simulink model "estimExp"  (R2017a)
settings: Solver=FixedStepDiscrete  StartTime=0.0  StopTime=20  FixedStep=prms.Ts  RelTol=1e-3
undefined symbols (not defined in the file or in its folder): prms
libraries: raspi_library x5, simulink x2
settings Model: SimulationMode=external  Creator=The MathWorks Inc.  LastModifiedBy=marti
settings SolverCC: PositivePriorityOrder=on
settings DataIOCC: LimitDataPoints=on  SaveFormat=Array
settings OptimizationCC: BlockReduction=off  BooleanDataType=off  DefaultUnderspecifiedDataType=single  LifeSpan=inf  MaxStackSize=64
settings DebuggingCC: SaveWithParameterizedLinksMsg=none  UnderspecifiedInitializationDetection=Classic  MergeDetectMultiDrivingBlocksExec=none  SignalResolutionControl=TryResolveAllWithWarning  InheritedTsInSrcMsg=error  ParameterTunabilityLossMsg=error  SFUnexpectedBacktrackingDiag=warning  SFNoUnconditionalDefaultTransitionDiag=warning  SFExecutionAtInitializationDiag=none
settings HardwareCC: ProdBitPerPointer=32  ProdBitPerSizeT=32  ProdBitPerPtrDiffT=32  ProdLargestAtomicInteger=Long  ProdLargestAtomicFloat=Double  ProdWordSize=32  ProdHWDeviceType=ARM Compatible->ARM Cortex
settings ModelReferenceCC: PropagateSignalLabelsOutOfModel=off
settings SFSimCC: MATLABDynamicMemAlloc=off
settings RTWCC: SystemTargetFile=ert.tlc  HardwareBoard=Raspberry Pi  TLCOptions=-aInlineSetEventsForThisBaseRateFcn=TLC_FALSE -aSuppressMultiTaskScheduler=TLC_FALSE -aRateBasedStepFcn=0  TemplateMakefile=ert_default_tmf  Description=Embedded Coder  GenerateReport=on  RTWVerbose=off  Toolchain=GNU GCC Raspberry Pi  BuildConfiguration=Specify  IncludeHyperlinkInReport=on  GenerateTraceInfo=on  GenerateTraceReport=on  GenerateTraceReportSl=on  GenerateTraceReportSf=on  GenerateTraceReportEml=on
settings CodeAppCC: ForceParamTrailComments=on  IgnoreCustomStorageClasses=off  OperatorAnnotations=on  SimulinkDataObjDesc=on  SFDataObjDesc=on  MATLABFcnDesc=on  MangleLength=10  InsertBlockDesc=on  MATLABSourceComments=on
settings ERTTargetCC: MultiwordLength=2048  SupportContinuousTime=on  SupportVariableSizeSignals=on
settings ConfigComp: CovMetricSettings=dw  CovHtmlReporting=on  CovSaveCumulativeToWorkspaceVar=on  CovSaveSingleToWorkspaceVar=on  CovExternalEMLEnable=off  CovSFcnEnable=off

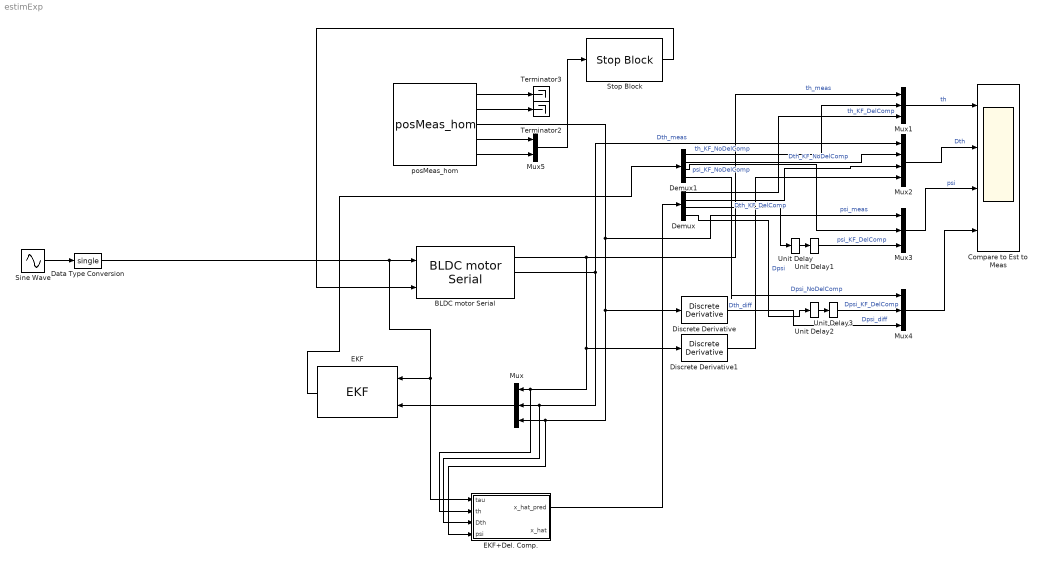
== system estimExp ==
  BLDC motor Serial : raspi_library/BLDC motor Serial  sampleTime=prms.Ts
  Compare to Est to Meas : Scope  NumInputPorts=4
  Data Type Conversion : DataTypeConversion  OutDataTypeStr=single
  Demux : Demux
  Demux1 : Demux
  Discrete Derivative : simulink/Discrete/Discrete Derivative  gainval=1.0  ICPrevScaledInput=0.0  OutMin=[]  OutMax=[]  OutDataType=fixdt(1, 16)  OutScaling=2^-10  DoSatur=off
  Discrete Derivative1 : simulink/Discrete/Discrete Derivative  gainval=1.0  ICPrevScaledInput=0.0  OutMin=[]  OutMax=[]  OutDataType=fixdt(1, 16)  OutScaling=2^-10  DoSatur=off
  EKF : raspi_library/EKF
  EKF+Del. Comp. : Subsystem
  Mux{,1,3..4} (4 alike) : Mux  Inputs=3
  Mux2 : Mux
  Mux5 : Mux  Inputs=2
  Sine Wave : Sin  Amplitude=0.05  Frequency=2*pi  SampleTime=prms.Ts
  Stop Block : raspi_library/Stop Block
  Terminator2 : Terminator
  Terminator3 : Terminator
  Unit Delay{,1..3} (4 alike) : UnitDelay  SampleTime=-1
  posMeas_hom : raspi_library/posMeas_hom  H=H  sampleTime=prms.Ts
  wires:
  posMeas_hom/5 -> Mux5/2
  posMeas_hom/4 -> Mux5/1
  posMeas_hom/2 -> Terminator2/1
  posMeas_hom/1 -> Terminator3/1
  posMeas_hom/3 -> Mux3/1, Discrete Derivative/1, EKF+Del. Comp./4(psi), Mux/3  "psi_meas"
  Mux/1 -> EKF/2
  BLDC motor Serial/1 -> Discrete Derivative1/1, EKF+Del. Comp./2(th), Mux/1, Mux1/1  "th_meas"
  BLDC motor Serial/2 -> EKF+Del. Comp./3(Dth), Mux/2, Mux2/1  "Dth_meas"
  EKF/1 -> Demux1/1
  Mux2/1 -> Compare to Est to Meas/2  "Dth"
  Mux3/1 -> Compare to Est to Meas/3  "psi"
  Mux1/1 -> Compare to Est to Meas/1  "th"
  Mux4/1 -> Compare to Est to Meas/4
  Mux5/1 -> Stop Block/1
  Stop Block/1 -> BLDC motor Serial/2
  Sine Wave/1 -> Data Type Conversion/1
  Data Type Conversion/1 -> EKF+Del. Comp./1(tau), EKF/1, BLDC motor Serial/1
  EKF+Del. Comp./1(x_hat_pred) -> Demux/1
  Demux/1 -> Mux1/3  "th_KF_DelComp"
  Demux1/1 -> Mux1/2  "th_KF_NoDelComp"
  Demux1/2 -> Mux2/2  "Dth_KF_NoDelComp"
  Demux/2 -> Mux2/3  "Dth_KF_DelComp"
  Demux1/3 -> Mux3/2  "psi_KF_NoDelComp"
  Demux/3 -> Unit Delay/1
  Unit Delay/1 -> Unit Delay1/1
  Unit Delay1/1 -> Mux3/3  "psi_KF_DelComp"
  Discrete Derivative1/1 -> Mux2/4  "Dth_diff"
  Discrete Derivative/1 -> Mux4/3  "Dpsi_diff"
  Unit Delay3/1 -> Mux4/2  "Dpsi_KF_DelComp"
  Unit Delay2/1 -> Unit Delay3/1
  Demux/4 -> Unit Delay2/1  "Dpsi"
  Demux1/4 -> Mux4/1  "Dpsi_NoDelComp"

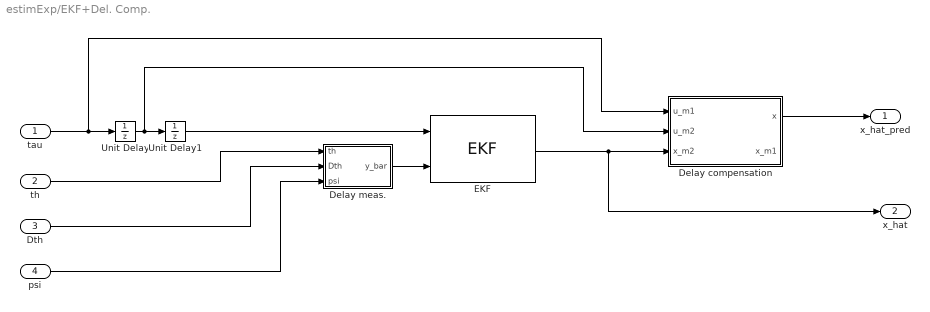
== system estimExp/EKF+Del. Comp. ==
  tau : Inport
  th : Inport  Port=2
  Dth : Inport  Port=3
  psi : Inport  Port=4
  Delay compensation : Subsystem
  Delay meas. : Subsystem
  EKF : raspi_library/EKF
  Unit Delay : UnitDelay  SampleTime=-1
  Unit Delay1 : UnitDelay  SampleTime=-1
  x_hat_pred : Outport
  x_hat : Outport  Port=2
  wires:
  Delay meas./1(y_bar) -> EKF/2
  Delay compensation/1(x) -> x_hat_pred/1
  EKF/1 -> x_hat/1, Delay compensation/3(x_m2)
  th/1 -> Delay meas./1(th)
  Dth/1 -> Delay meas./2(Dth)
  psi/1 -> Delay meas./3(psi)
  tau/1 -> Delay compensation/1(u_m1), Unit Delay/1
  Unit Delay1/1 -> EKF/1
  Unit Delay/1 -> Delay compensation/2(u_m2), Unit Delay1/1

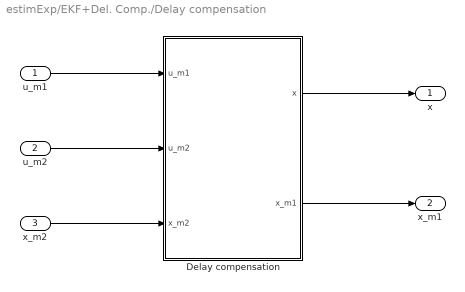
== system estimExp/EKF+Del. Comp./Delay compensation ==
  u_m1 : Inport
  u_m2 : Inport  Port=2
  x_m2 : Inport  Port=3
  Delay compensation : MATLAB Function  TreatAsAtomicUnit=on  SystemSampleTime=prms.Ts
  x : Outport
  x_m1 : Outport  Port=2
  wires:
  x_m2/1 -> Delay compensation/3(x_m2)
  u_m1/1 -> Delay compensation/1(u_m1)
  u_m2/1 -> Delay compensation/2(u_m2)
  Delay compensation/1(x) -> x/1
  Delay compensation/2(x_m1) -> x_m1/1

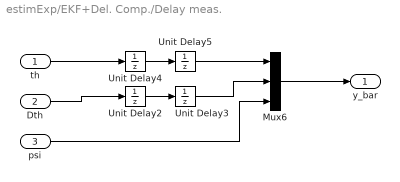
== system estimExp/EKF+Del. Comp./Delay meas. ==
  th : Inport
  Dth : Inport  Port=2
  psi : Inport  Port=3
  Mux6 : Mux  Inputs=3
  Unit Delay{2..5} (4 alike) : UnitDelay  SampleTime=-1
  y_bar : Outport
  wires:
  Unit Delay5/1 -> Mux6/1
  Mux6/1 -> y_bar/1
  Unit Delay2/1 -> Unit Delay3/1
  Unit Delay3/1 -> Mux6/2
  Unit Delay4/1 -> Unit Delay5/1
  th/1 -> Unit Delay4/1
  Dth/1 -> Unit Delay2/1
  psi/1 -> Mux6/3

== matlab function estimExp/EKF+Del. Comp./Delay compensation/Delay compensation ==
  data: u_m1 input; u_m2 input; x output; x_m2 input; prms parameter; x_m1 output
function [x, x_m1] = delayCompensation( u_m1, u_m2, x_m2, prms)

N = 1;
T = prms.Ts/N;

% Time Update - 1
x_old = x_m2;
x_new = single(zeros(4,1));
for i = 1:N
    x_new = x_old + T*ballInAHoopODEFUN(0, x_old, prms, u_m2);
    x_old = x_new;
end
x_m1 = x_new;

% Time Update - 2
x_old = x_m1;
x_new = single(zeros(4,1));
for i = 1:N
    x_new = x_old + T*ballInAHoopODEFUN(0, x_old, prms, u_m1);
    x_old = x_new;
end
x = x_new;
